simulink model "Example_Simulink_MagicFormulaTyre"  (R2021a)
settings: Solver=FixedStepDiscrete  StartTime=0.0  StopTime=0.4  FixedStep=0.01  RelTol=1e-3
libraries: MagicFormulaTyreLibrary x1, simulink x1
settings Model: Creator=Tom  LastModifiedBy=Tom

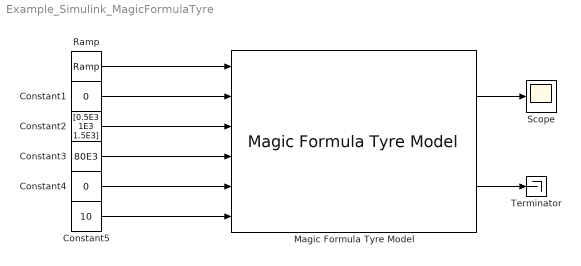
== system Example_Simulink_MagicFormulaTyre ==
  Constant1 : Constant  Value=0
  Constant2 : Constant  Value=[0.5E3 1E3 1.5E3]
  Constant3 : Constant  Value=80E3
  Constant4 : Constant  Value=0
  Constant5 : Constant  Value=10
  Magic Formula Tyre Model : MagicFormulaTyreLibrary/Magic Formula Tyre Model  file='doc/examples/fsae-ttc-data/fsaettc_obfuscated.tir'  sideText=Left  version=MagicFormulaVersion.v61
      settings: SourceProductName=Magic Formula Tyre Library
  Ramp : simulink/Sources/Ramp  slope=1  start=0  InitialOutput=-0.2
  Scope : Scope
  Terminator : Terminator
  wires:
  Ramp/1 -> Magic Formula Tyre Model/1
  Constant1/1 -> Magic Formula Tyre Model/2
  Constant3/1 -> Magic Formula Tyre Model/4
  Constant4/1 -> Magic Formula Tyre Model/5
  Magic Formula Tyre Model/1 -> Scope/1
  Magic Formula Tyre Model/2 -> Terminator/1
  Constant2/1 -> Magic Formula Tyre Model/3
  Constant5/1 -> Magic Formula Tyre Model/6
